simulink model "T1"  (R2025b)
settings: Solver=VariableStepAuto  StartTime=0.0  StopTime=10.0  RelTol=1e-3
settings Model: Creator=yunzhuorui  LastModifiedBy=yunzhuorui

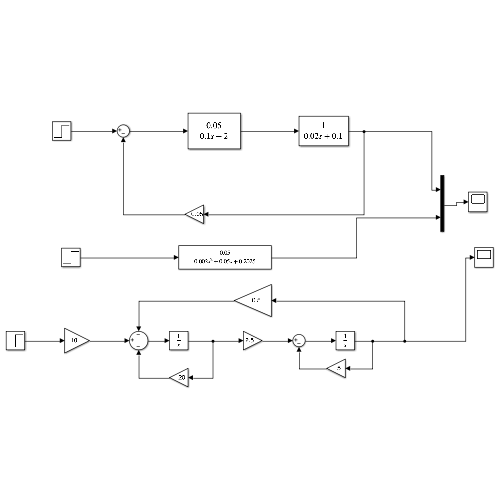
[thumbnail: Simulink's stored preview of the top-level diagram]
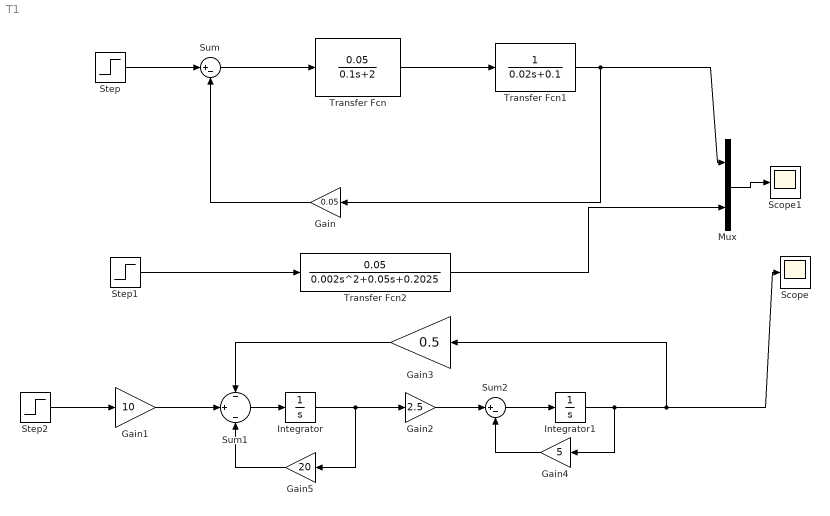
== system T1 ==
  Gain : Gain  Gain=0.05
  Gain1 : Gain  Gain=10
  Gain2 : Gain  Gain=2.5
  Gain3 : Gain  Gain=0.5
  Gain4 : Gain  Gain=5
  Gain5 : Gain  Gain=20
  Integrator : Integrator
  Integrator1 : Integrator
  Mux : Mux  Inputs=2
  Scope : Scope
      settings: ActiveDisplayYMinimum=-521632.1688956772  ActiveDisplayYMaximum=1.8800320748448954E+6
  Scope1 : Scope
      settings: ActiveDisplayYMinimum=-1  ActiveDisplayYMaximum=1
  Step : Step  SampleTime=0
  Step1 : Step  SampleTime=0
  Step2 : Step  SampleTime=0
  Sum : Sum  Inputs=|+-
  Sum1 : Sum  Inputs=-|+|-
  Sum2 : Sum  Inputs=|+-
  Transfer Fcn : TransferFcn  Numerator=[0.05]  Denominator=[0.1 2]
  Transfer Fcn1 : TransferFcn  Denominator=[0.02 0.1]
  Transfer Fcn2 : TransferFcn  Numerator=[0.05]  Denominator=[0.002 0.05 0.2025]
  wires:
  Step/1 -> Sum/1
  Sum/1 -> Transfer Fcn/1
  Transfer Fcn/1 -> Transfer Fcn1/1
  Gain/1 -> Sum/2
  Step1/1 -> Transfer Fcn2/1
  Sum1/1 -> Integrator/1
  Integrator/1 -> Gain5/1, Gain2/1
  Gain2/1 -> Sum2/1
  Sum2/1 -> Integrator1/1
  Gain4/1 -> Sum2/2
  Gain5/1 -> Sum1/3
  Transfer Fcn1/1 -> Gain/1, Mux/1
  Transfer Fcn2/1 -> Mux/2
  Gain3/1 -> Sum1/1
  Gain1/1 -> Sum1/2
  Integrator1/1 -> Gain4/1, Gain3/1, Scope/1
  Step2/1 -> Gain1/1
  Mux/1 -> Scope1/1
